simulink model "rotations_test"  (R2023b)
settings: Solver=VariableStepAuto  StartTime=0.0  StopTime=10.0  RelTol=1e-3
undefined symbols (not defined in the file): phi, psi, theta
libraries: dyn_lib x4
settings Model: Creator=brent  LastModifiedBy=brent

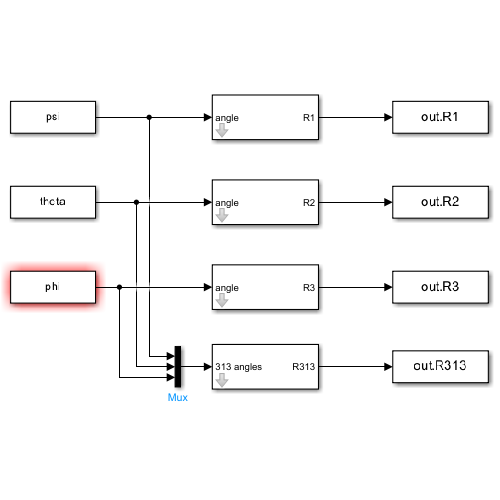
[thumbnail: Simulink's stored preview of the top-level diagram]
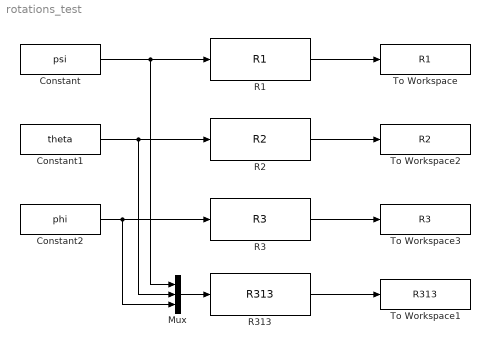
== system rotations_test ==
  Constant : Constant  Value=psi
  Constant1 : Constant  Value=theta
  Constant2 : Constant  Value=phi
  Mux : Mux  Inputs=3
  R1 : dyn_lib/R1
      settings: SourceProductName=Dynamics library
  R2 : dyn_lib/R2
      settings: SourceProductName=Dynamics library
  R3 : dyn_lib/R3
      settings: SourceProductName=Dynamics library
  R313 : dyn_lib/R313
      settings: SourceProductName=Dynamics library
  To Workspace : ToWorkspace  VariableName=R1  SaveFormat=Structure  SampleTime=-1
      settings: Save2DSignal=2-D array (concatenate along first dimension)
  To Workspace1 : ToWorkspace  VariableName=R313  SaveFormat=Structure  SampleTime=-1
      settings: Save2DSignal=2-D array (concatenate along first dimension)
  To Workspace2 : ToWorkspace  VariableName=R2  SaveFormat=Structure  SampleTime=-1
      settings: Save2DSignal=2-D array (concatenate along first dimension)
  To Workspace3 : ToWorkspace  VariableName=R3  SaveFormat=Structure  SampleTime=-1
      settings: Save2DSignal=2-D array (concatenate along first dimension)
  wires:
  Constant/1 -> Mux/1, R1/1
  Constant1/1 -> Mux/2, R2/1
  Constant2/1 -> Mux/3, R3/1
  Mux/1 -> R313/1
  R1/1 -> To Workspace/1
  R2/1 -> To Workspace2/1
  R3/1 -> To Workspace3/1
  R313/1 -> To Workspace1/1
